simulink library "battery_lib_2011"  (Simulink 7.8)
settings: Solver=ode45  StartTime=0.0  StopTime=10.0  RelTol=1e-3
values from neighbouring files (symbols this model uses):
  Tds = Ts    (= 8e-05)    [global_parameters.m]
undefined symbols (not defined in the file or in its folder): DiscIntNeverNeededParam
libraries: simulink x1
settings Model: Creator=CH24070  LastModifiedBy=ma25949

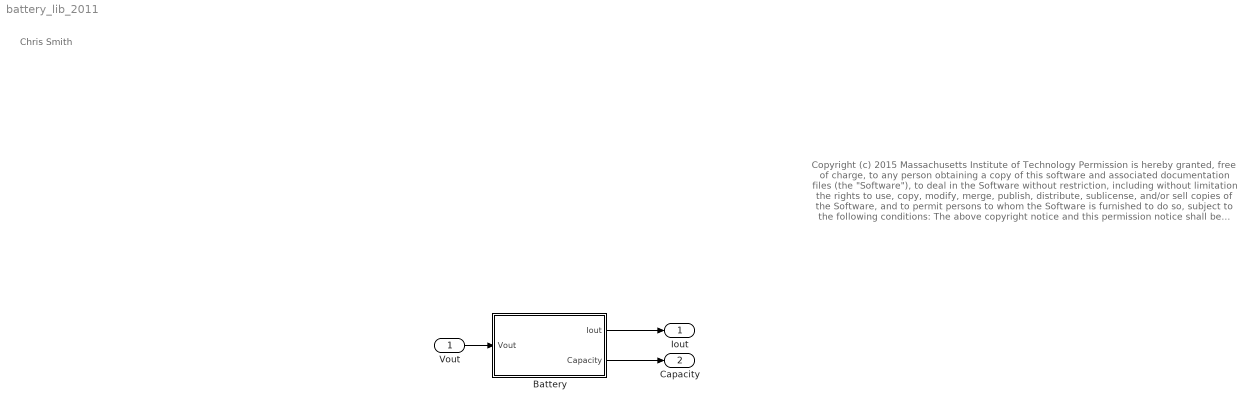
== system battery_lib_2011 ==
  note: Chris Smith
  note: Copyright (c) 2015 Massachusetts Institute of Technology
      | Permission is hereby granted, free of charge, to any person obtaining a copy of this software and associated documentation files (the "Software"), to deal in the Software without restriction, including without limitation the rights to use, copy, modify, merge, publish, distribute, sublicense, and/or sell copies of the Software, and to permit persons to whom the Software is furnished to do so, subject to the following conditions:
      |
      | The above copyright notice and this permission notice shall be included in all copies or substantial portions of the Software.
      |
      | THE SOFTWARE IS PROVIDED "AS IS", WITHOUT WARRANTY OF ANY KIND, EXPRESS OR IMPLIED, INCLUDING BUT NOT LIMITED TO THE WARRANTIES OF MERCHANTABILITY, FITNESS FOR A PARTICULAR PURPOSE AND NONINFRINGEMENT. IN NO EVENT SHALL THE AUTHORS OR COPYRIGHT HOLDERS BE LIABLE FOR ANY CLAIM,
      | DAMAGES OR OTHER LIABILITY, WHETHER IN AN ACTION OF CONTRACT, TORT OR OTHERWISE, ARISING FROM, OUT OF OR IN CONNECTION WITH THE SOFTWARE OR THE USE OR OTHER DEALINGS IN THE SOFTWARE.
  Vout : Inport
  Battery : Subsystem  mask(Very simple battery model.  ){energy=5000, esr=0.01, Vdc_nom=1200}
      mask prompts: energy "Capacity  (kWh)"; esr "Output Resistance (Ohms)"; Vdc_nom "Open Circuit Voltage"
      mask help: Model integrates charge and stops at the rated capacity. When charge is all removed the current drops to zero.
      mask Help: This model views the battery as a voltage source with a fixed equivalent series resistance and a perfect integrator for capacity.
  Iout : Outport
  Capacity : Outport  Port=2
  wires:
  Vout/1 -> Battery/1(Vout)
  Battery/1(Iout) -> Iout/1
  Battery/2(Capacity) -> Capacity/1

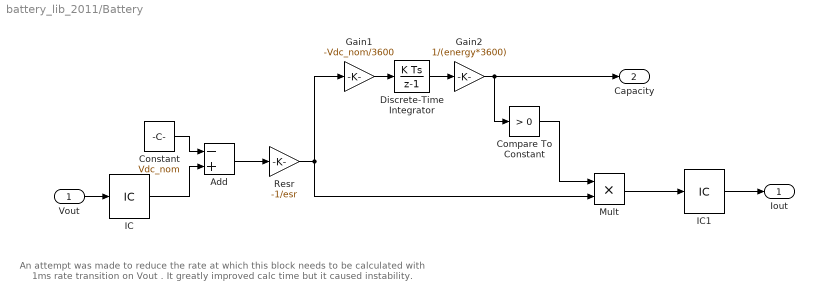
== system battery_lib_2011/Battery ==
  note: An attempt was made to reduce the rate at which this block
      | needs to be calculated with 1ms rate transition on
      | Vout .  It greatly improved calc time but it caused instability.
  Vout : Inport
  Add : Sum  Inputs=-+
  Compare To Constant : simulink/Logic and Bit Operations/Compare To Constant  relop=>  const=0  OutDataTypeStr=uint8
  Constant : Constant  Value=Vdc_nom  SampleTime=Tds
  Discrete-Time Integrator : DiscreteIntegrator  InitialCondition=energy*3600*0.5  InitialConditionMode=State only (most efficient)  SampleTime=Tds  LimitOutput=on  UpperSaturationLimit=energy*3600  LowerSaturationLimit=0  ICPrevOutput=DiscIntNeverNeededParam  ICPrevScaledInput=DiscIntNeverNeededParam
  Gain1 : Gain  Gain=-Vdc_nom/3600
  Gain2 : Gain  Gain=1/(energy*3600)
  IC : InitialCondition  Value=Vdc_nom
  IC1 : InitialCondition  Value=0
  Mult : Product  Inputs=**
  Resr : Gain  Gain=-1/esr
  Iout : Outport
  Capacity : Outport  Port=2
  wires:
  Constant/1 -> Add/1
  Add/1 -> Resr/1
  Gain1/1 -> Discrete-Time Integrator/1
  Compare To Constant/1 -> Mult/1
  Vout/1 -> IC/1
  Mult/1 -> IC1/1
  Resr/1 -> Mult/2, Gain1/1
  Gain2/1 -> Capacity/1, Compare To Constant/1
  Discrete-Time Integrator/1 -> Gain2/1
  IC/1 -> Add/2
  IC1/1 -> Iout/1
